simulink model "ScriptDemo"  (R2022b)
settings: configuration reference "TmVcThermal_Configuration_sub" (kept outside this file)
undefined symbols (not defined in the file or in its folder): aaaa, bbbb, cTmComprCtrl_D_u8HvacFlowTable_db, cTmComprCtrl_D_u8HvacFlowTable_sw, cTmComprCtrl_n_i16ChillCmpIMax, cTmComprCtrl_n_i16ChillCmpIMin, cTmComprCtrl_n_i16ChillCmpIMin666, cTmComprCtrl_n_i16ChillCmpPMax, cTmComprCtrl_n_i16ChillCmpPMin, cTmComprCtrl_n_i16CmpChillCoolRpmKiMax, cTmComprCtrl_n_i16CmpChillCoolRpmKiMin, cTmComprCtrl_n_i16CmpChillCoolRpmKpMax, cTmComprCtrl_n_i16CmpChillCoolRpmKpMin, cTmComprCtrl_n_i16CmpCoolRpmKiMax, cTmComprCtrl_n_i16CmpCoolRpmKiMin, cTmComprCtrl_n_i16CmpCoolRpmKpMax, cTmComprCtrl_n_i16CmpCoolRpmKpMin, cTmComprCtrl_n_i16SM4CmpHeatKiMax, cTmComprCtrl_n_i16SM4CmpHeatKiMin, cTmComprCtrl_n_i16SM4CmpHeatKpMax, cTmComprCtrl_n_i16SM4CmpHeatKpMin, cTmComprCtrl_n_i16SM5CmpHeatKiMax, cTmComprCtrl_n_i16SM5CmpHeatKiMin, cTmComprCtrl_n_i16SM5CmpHeatKpMax, cTmComprCtrl_n_i16SM5CmpHeatKpMin, cTmComprCtrl_n_i16SM6CmpHeatKiMax, cTmComprCtrl_n_i16SM6CmpHeatKiMin, cTmComprCtrl_n_i16SM6CmpHeatKpMax, cTmComprCtrl_n_i16SM6CmpHeatKpMin, cTmComprCtrl_n_u16CmpMaxSpdFanFltLimt, cTmComprCtrl_n_u16CmpMaxSpdLoSidePFltLimt, cTmComprCtrl_n_u16CmpMaxSpdSensorFltLimt, cTmComprCtrl_n_u16CompMinRpm, cTmComprCtrl_n_u16CompRpmIncThres, cTmComprCtrl_t_u16BattCooltFFPeriod, cTmComprCtrl_t_u16BattCooltPIPeriod, cTmComprCtrl_t_u16CmpCoolFFPeriod, cTmComprCtrl_t_u16CmpCoolPIPeriod, cTmComprCtrl_t_u16CoolCmpChillFFPeriod, cTmComprCtrl_t_u16CoolCmpChillPIPeriod, cTmComprCtrl_t_u16SM4CmpHeatFFPeriod, cTmComprCtrl_t_u16SM4CmpHeatPIPeriod, cTmComprCtrl_t_u16SM5CmpHeatFFPeriod, cTmComprCtrl_t_u16SM5CmpHeatPIPeriod, cTmComprCtrl_t_u16SM6CmpHeatFFPeriod, cTmComprCtrl_t_u16SM6CmpHeatPIPeriod, cTmComprCtrl_Te_EvapClearInteg, cTmComprCtrl_Te_i16HpReqTempSaturoffset, cTmComprCtrl_Te_i16SatLpReplaceDiff, cTmComprCtrl_Te_i16SM3BatDiffStartEvapDecOffset, cTmComprCtrl_Te_i16SM3EvapLo, cTmComprCtrl_Te_i16SM3TBatDiffEntEvapDecOffset, cTmComprCtrl_Te_i16SM3TBatDiffEntEvapDecOffsetQuit, cTmComprCtrl_Te_s32ErrCmpChillPIContinueCoolH, cTmComprCtrl_Te_s32ErrCmpChillPIContinueCoolL, cTmComprCtrl_Te_s32ErrCmpPIContinueChillH, cTmComprCtrl_Te_s32ErrCmpPIContinueChillL, cTmComprCtrl_Te_s32ErrCmpPIContinueCoolH, cTmComprCtrl_Te_s32ErrCmpPIContinueCoolL, cTmComprCtrl_Te_s32ErrCmpPIContinueHeatH ... (+398)
libraries: simulink x846, PCMULib x711, simulink_need_slupdate x4
(part 12 of 49)

== system ScriptDemo/Create/createSigOnLine/Before3 ==
  sTmRefriVlvCtrl_X_s32CEXVPosReqIn : Inport  OutDataTypeStr=single  OutputFunctionCall=on
  sTmRefriVlvCtrl_X_s32EEXVPosReqIn : Inport  Port=2  OutDataTypeStr=single
  sTmRefriVlvCtrl_X_s32BEXVPosReqIn : Inport  Port=3  OutDataTypeStr=single
  yTmRefriVlvCtrl_B_HpcCexvMovEnableIn : Inport  Port=4  OutDataTypeStr=boolean
  sTmRefriVlvCtrl_Z_u8CEXVInitStateIn : Inport  Port=5  OutDataTypeStr=uint8
  yTmRefriVlvCtrl_B_CexvCalibReqIn : Inport  Port=6  OutDataTypeStr=boolean
  yTmRefriVlvCtrl_B_HpcEexvMovEnableIn : Inport  Port=7  OutDataTypeStr=boolean
  sTmRefriVlvCtrl_Z_u8EEXVInitStateIn : Inport  Port=8  OutDataTypeStr=uint8
  yTmRefriVlvCtrl_B_EexvCalibReqIn : Inport  Port=9  OutDataTypeStr=boolean
  yTmRefriVlvCtrl_B_HpcBexvMovEnableIn : Inport  Port=10  OutDataTypeStr=boolean
  sTmRefriVlvCtrl_Z_u8BEXVInitStateIn : Inport  Port=11  OutDataTypeStr=uint8
  yTmRefriVlvCtrl_B_BexvCalibReqIn : Inport  Port=12  OutDataTypeStr=boolean
  sTmRefriVlvCtrl_X_s32SM3BexvMaxPosIn : Inport  Port=13  OutDataTypeStr=single
  yTmRefriVlvCtrl_B_EvapBattTLimBexvEnaIn : Inport  Port=14  OutDataTypeStr=boolean
  sTmRefriVlvCtrl_D_u8EexvRefriSwitchStIn : Inport  Port=15  OutDataTypeStr=uint8
  sTmRefriVlvCtrl_D_u8CexvRefriSwitchStIn : Inport  Port=16  OutDataTypeStr=uint8
  sTmRefriVlvCtrl_D_u8BexvRefriSwitchStIn : Inport  Port=17  OutDataTypeStr=uint8
  Before : Subsystem
  sTmRefriVlvCtrl_X_s32CEXVPosReq : Outport  OutDataTypeStr=single
  sTmRefriVlvCtrl_X_s32EEXVPosReq : Outport  Port=2  OutDataTypeStr=single
  sTmRefriVlvCtrl_X_s32BEXVPosReq : Outport  Port=3  OutDataTypeStr=single
  yTmRefriVlvCtrl_B_HpcCexvMovEnable : Outport  Port=4  OutDataTypeStr=boolean
  sTmRefriVlvCtrl_Z_u8CEXVInitState : Outport  Port=5  OutDataTypeStr=uint8
  yTmRefriVlvCtrl_B_CexvCalibReq : Outport  Port=6  OutDataTypeStr=boolean
  yTmRefriVlvCtrl_B_HpcEexvMovEnable : Outport  Port=7  OutDataTypeStr=boolean
  sTmRefriVlvCtrl_Z_u8EEXVInitState : Outport  Port=8  OutDataTypeStr=uint8
  yTmRefriVlvCtrl_B_EexvCalibReq : Outport  Port=9  OutDataTypeStr=boolean
  yTmRefriVlvCtrl_B_HpcBexvMovEnable : Outport  Port=10  OutDataTypeStr=boolean
  sTmRefriVlvCtrl_Z_u8BEXVInitState : Outport  Port=11  OutDataTypeStr=uint8
  yTmRefriVlvCtrl_B_BexvCalibReq : Outport  Port=12  OutDataTypeStr=boolean
  sTmRefriVlvCtrl_X_s32SM3BexvMaxPos : Outport  Port=13  OutDataTypeStr=single
  yTmRefriVlvCtrl_B_EvapBattTLimBexvEna : Outport  Port=14  OutDataTypeStr=boolean
  sTmRefriVlvCtrl_D_u8EexvRefriSwitchSt : Outport  Port=15  OutDataTypeStr=uint8
  sTmRefriVlvCtrl_D_u8CexvRefriSwitchSt : Outport  Port=16  OutDataTypeStr=uint8
  sTmRefriVlvCtrl_D_u8BexvRefriSwitchSt : Outport  Port=17  OutDataTypeStr=uint8
  wires:
  sTmRefriVlvCtrl_X_s32CEXVPosReqIn/1 -> Before/1(sTmRefriVlvCtrl_X_s32CEXVPosReqIn)
  sTmRefriVlvCtrl_X_s32EEXVPosReqIn/1 -> Before/2(sTmRefriVlvCtrl_X_s32EEXVPosReqIn)
  sTmRefriVlvCtrl_X_s32BEXVPosReqIn/1 -> Before/3(sTmRefriVlvCtrl_X_s32BEXVPosReqIn)
  yTmRefriVlvCtrl_B_HpcCexvMovEnableIn/1 -> Before/4(yTmRefriVlvCtrl_B_HpcCexvMovEnableIn)
  sTmRefriVlvCtrl_Z_u8CEXVInitStateIn/1 -> Before/5(sTmRefriVlvCtrl_Z_u8CEXVInitStateIn)
  yTmRefriVlvCtrl_B_CexvCalibReqIn/1 -> Before/6(yTmRefriVlvCtrl_B_CexvCalibReqIn)
  yTmRefriVlvCtrl_B_HpcEexvMovEnableIn/1 -> Before/7(yTmRefriVlvCtrl_B_HpcEexvMovEnableIn)
  sTmRefriVlvCtrl_Z_u8EEXVInitStateIn/1 -> Before/8(sTmRefriVlvCtrl_Z_u8EEXVInitStateIn)
  yTmRefriVlvCtrl_B_EexvCalibReqIn/1 -> Before/9(yTmRefriVlvCtrl_B_EexvCalibReqIn)
  yTmRefriVlvCtrl_B_HpcBexvMovEnableIn/1 -> Before/10(yTmRefriVlvCtrl_B_HpcBexvMovEnableIn)
  sTmRefriVlvCtrl_Z_u8BEXVInitStateIn/1 -> Before/11(sTmRefriVlvCtrl_Z_u8BEXVInitStateIn)
  yTmRefriVlvCtrl_B_BexvCalibReqIn/1 -> Before/12(yTmRefriVlvCtrl_B_BexvCalibReqIn)
  sTmRefriVlvCtrl_X_s32SM3BexvMaxPosIn/1 -> Before/13(sTmRefriVlvCtrl_X_s32SM3BexvMaxPosIn)
  yTmRefriVlvCtrl_B_EvapBattTLimBexvEnaIn/1 -> Before/14(yTmRefriVlvCtrl_B_EvapBattTLimBexvEnaIn)
  sTmRefriVlvCtrl_D_u8EexvRefriSwitchStIn/1 -> Before/15(sTmRefriVlvCtrl_D_u8EexvRefriSwitchStIn)
  sTmRefriVlvCtrl_D_u8CexvRefriSwitchStIn/1 -> Before/16(sTmRefriVlvCtrl_D_u8CexvRefriSwitchStIn)
  sTmRefriVlvCtrl_D_u8BexvRefriSwitchStIn/1 -> Before/17(sTmRefriVlvCtrl_D_u8BexvRefriSwitchStIn)
  Before/1(sTmRefriVlvCtrl_X_s32CEXVPosReq) -> sTmRefriVlvCtrl_X_s32CEXVPosReq/1
  Before/2(sTmRefriVlvCtrl_X_s32EEXVPosReq) -> sTmRefriVlvCtrl_X_s32EEXVPosReq/1
  Before/3(sTmRefriVlvCtrl_X_s32BEXVPosReq) -> sTmRefriVlvCtrl_X_s32BEXVPosReq/1
  Before/4(yTmRefriVlvCtrl_B_HpcCexvMovEnable) -> yTmRefriVlvCtrl_B_HpcCexvMovEnable/1
  Before/5(sTmRefriVlvCtrl_Z_u8CEXVInitState) -> sTmRefriVlvCtrl_Z_u8CEXVInitState/1
  Before/6(yTmRefriVlvCtrl_B_CexvCalibReq) -> yTmRefriVlvCtrl_B_CexvCalibReq/1
  Before/7(yTmRefriVlvCtrl_B_HpcEexvMovEnable) -> yTmRefriVlvCtrl_B_HpcEexvMovEnable/1
  Before/8(sTmRefriVlvCtrl_Z_u8EEXVInitState) -> sTmRefriVlvCtrl_Z_u8EEXVInitState/1
  Before/9(yTmRefriVlvCtrl_B_EexvCalibReq) -> yTmRefriVlvCtrl_B_EexvCalibReq/1
  Before/10(yTmRefriVlvCtrl_B_HpcBexvMovEnable) -> yTmRefriVlvCtrl_B_HpcBexvMovEnable/1
  Before/11(sTmRefriVlvCtrl_Z_u8BEXVInitState) -> sTmRefriVlvCtrl_Z_u8BEXVInitState/1
  Before/12(yTmRefriVlvCtrl_B_BexvCalibReq) -> yTmRefriVlvCtrl_B_BexvCalibReq/1
  Before/13(sTmRefriVlvCtrl_X_s32SM3BexvMaxPos) -> sTmRefriVlvCtrl_X_s32SM3BexvMaxPos/1
  Before/14(yTmRefriVlvCtrl_B_EvapBattTLimBexvEna) -> yTmRefriVlvCtrl_B_EvapBattTLimBexvEna/1
  Before/15(sTmRefriVlvCtrl_D_u8EexvRefriSwitchSt) -> sTmRefriVlvCtrl_D_u8EexvRefriSwitchSt/1
  Before/16(sTmRefriVlvCtrl_D_u8CexvRefriSwitchSt) -> sTmRefriVlvCtrl_D_u8CexvRefriSwitchSt/1
  Before/17(sTmRefriVlvCtrl_D_u8BexvRefriSwitchSt) -> sTmRefriVlvCtrl_D_u8BexvRefriSwitchSt/1

== system ScriptDemo/Create/createSigOnLine/Before4 ==
  sTmRefriVlvCtrl_X_s32CEXVPosReqIn : Inport  OutDataTypeStr=single  OutputFunctionCall=on
  sTmRefriVlvCtrl_X_s32EEXVPosReqIn : Inport  Port=2  OutDataTypeStr=single
  sTmRefriVlvCtrl_X_s32BEXVPosReqIn : Inport  Port=3  OutDataTypeStr=single
  yTmRefriVlvCtrl_B_HpcCexvMovEnableIn : Inport  Port=4  OutDataTypeStr=boolean
  sTmRefriVlvCtrl_Z_u8CEXVInitStateIn : Inport  Port=5  OutDataTypeStr=uint8
  yTmRefriVlvCtrl_B_CexvCalibReqIn : Inport  Port=6  OutDataTypeStr=boolean
  yTmRefriVlvCtrl_B_HpcEexvMovEnableIn : Inport  Port=7  OutDataTypeStr=boolean
  sTmRefriVlvCtrl_Z_u8EEXVInitStateIn : Inport  Port=8  OutDataTypeStr=uint8
  yTmRefriVlvCtrl_B_EexvCalibReqIn : Inport  Port=9  OutDataTypeStr=boolean
  yTmRefriVlvCtrl_B_HpcBexvMovEnableIn : Inport  Port=10  OutDataTypeStr=boolean
  sTmRefriVlvCtrl_Z_u8BEXVInitStateIn : Inport  Port=11  OutDataTypeStr=uint8
  yTmRefriVlvCtrl_B_BexvCalibReqIn : Inport  Port=12  OutDataTypeStr=boolean
  sTmRefriVlvCtrl_X_s32SM3BexvMaxPosIn : Inport  Port=13  OutDataTypeStr=single
  yTmRefriVlvCtrl_B_EvapBattTLimBexvEnaIn : Inport  Port=14  OutDataTypeStr=boolean
  sTmRefriVlvCtrl_D_u8EexvRefriSwitchStIn : Inport  Port=15  OutDataTypeStr=uint8
  sTmRefriVlvCtrl_D_u8CexvRefriSwitchStIn : Inport  Port=16  OutDataTypeStr=uint8
  sTmRefriVlvCtrl_D_u8BexvRefriSwitchStIn : Inport  Port=17  OutDataTypeStr=uint8
  Before : Subsystem
  sTmRefriVlvCtrl_X_s32CEXVPosReq : Outport  OutDataTypeStr=single
  sTmRefriVlvCtrl_X_s32EEXVPosReq : Outport  Port=2  OutDataTypeStr=single
  sTmRefriVlvCtrl_X_s32BEXVPosReq : Outport  Port=3  OutDataTypeStr=single
  yTmRefriVlvCtrl_B_HpcCexvMovEnable : Outport  Port=4  OutDataTypeStr=boolean
  sTmRefriVlvCtrl_Z_u8CEXVInitState : Outport  Port=5  OutDataTypeStr=uint8
  yTmRefriVlvCtrl_B_CexvCalibReq : Outport  Port=6  OutDataTypeStr=boolean
  yTmRefriVlvCtrl_B_HpcEexvMovEnable : Outport  Port=7  OutDataTypeStr=boolean
  sTmRefriVlvCtrl_Z_u8EEXVInitState : Outport  Port=8  OutDataTypeStr=uint8
  yTmRefriVlvCtrl_B_EexvCalibReq : Outport  Port=9  OutDataTypeStr=boolean
  yTmRefriVlvCtrl_B_HpcBexvMovEnable : Outport  Port=10  OutDataTypeStr=boolean
  sTmRefriVlvCtrl_Z_u8BEXVInitState : Outport  Port=11  OutDataTypeStr=uint8
  yTmRefriVlvCtrl_B_BexvCalibReq : Outport  Port=12  OutDataTypeStr=boolean
  sTmRefriVlvCtrl_X_s32SM3BexvMaxPos : Outport  Port=13  OutDataTypeStr=single
  yTmRefriVlvCtrl_B_EvapBattTLimBexvEna : Outport  Port=14  OutDataTypeStr=boolean
  sTmRefriVlvCtrl_D_u8EexvRefriSwitchSt : Outport  Port=15  OutDataTypeStr=uint8
  sTmRefriVlvCtrl_D_u8CexvRefriSwitchSt : Outport  Port=16  OutDataTypeStr=uint8
  sTmRefriVlvCtrl_D_u8BexvRefriSwitchSt : Outport  Port=17  OutDataTypeStr=uint8
  wires:
  sTmRefriVlvCtrl_X_s32CEXVPosReqIn/1 -> Before/1(sTmRefriVlvCtrl_X_s32CEXVPosReqIn)  "sTmRefriVlvCtrl_X_s32CEXVPosReqIn"
  sTmRefriVlvCtrl_X_s32EEXVPosReqIn/1 -> Before/2(sTmRefriVlvCtrl_X_s32EEXVPosReqIn)  "sTmRefriVlvCtrl_X_s32EEXVPosReqIn"
  sTmRefriVlvCtrl_X_s32BEXVPosReqIn/1 -> Before/3(sTmRefriVlvCtrl_X_s32BEXVPosReqIn)  "sTmRefriVlvCtrl_X_s32BEXVPosReqIn"
  yTmRefriVlvCtrl_B_HpcCexvMovEnableIn/1 -> Before/4(yTmRefriVlvCtrl_B_HpcCexvMovEnableIn)  "yTmRefriVlvCtrl_B_HpcCexvMovEnableIn"
  sTmRefriVlvCtrl_Z_u8CEXVInitStateIn/1 -> Before/5(sTmRefriVlvCtrl_Z_u8CEXVInitStateIn)  "sTmRefriVlvCtrl_Z_u8CEXVInitStateIn"
  yTmRefriVlvCtrl_B_CexvCalibReqIn/1 -> Before/6(yTmRefriVlvCtrl_B_CexvCalibReqIn)  "yTmRefriVlvCtrl_B_CexvCalibReqIn"
  yTmRefriVlvCtrl_B_HpcEexvMovEnableIn/1 -> Before/7(yTmRefriVlvCtrl_B_HpcEexvMovEnableIn)  "yTmRefriVlvCtrl_B_HpcEexvMovEnableIn"
  sTmRefriVlvCtrl_Z_u8EEXVInitStateIn/1 -> Before/8(sTmRefriVlvCtrl_Z_u8EEXVInitStateIn)  "sTmRefriVlvCtrl_Z_u8EEXVInitStateIn"
  yTmRefriVlvCtrl_B_EexvCalibReqIn/1 -> Before/9(yTmRefriVlvCtrl_B_EexvCalibReqIn)  "yTmRefriVlvCtrl_B_EexvCalibReqIn"
  yTmRefriVlvCtrl_B_HpcBexvMovEnableIn/1 -> Before/10(yTmRefriVlvCtrl_B_HpcBexvMovEnableIn)  "yTmRefriVlvCtrl_B_HpcBexvMovEnableIn"
  sTmRefriVlvCtrl_Z_u8BEXVInitStateIn/1 -> Before/11(sTmRefriVlvCtrl_Z_u8BEXVInitStateIn)  "sTmRefriVlvCtrl_Z_u8BEXVInitStateIn"
  yTmRefriVlvCtrl_B_BexvCalibReqIn/1 -> Before/12(yTmRefriVlvCtrl_B_BexvCalibReqIn)  "yTmRefriVlvCtrl_B_BexvCalibReqIn"
  sTmRefriVlvCtrl_X_s32SM3BexvMaxPosIn/1 -> Before/13(sTmRefriVlvCtrl_X_s32SM3BexvMaxPosIn)  "sTmRefriVlvCtrl_X_s32SM3BexvMaxPosIn"
  yTmRefriVlvCtrl_B_EvapBattTLimBexvEnaIn/1 -> Before/14(yTmRefriVlvCtrl_B_EvapBattTLimBexvEnaIn)  "yTmRefriVlvCtrl_B_EvapBattTLimBexvEnaIn"
  sTmRefriVlvCtrl_D_u8EexvRefriSwitchStIn/1 -> Before/15(sTmRefriVlvCtrl_D_u8EexvRefriSwitchStIn)  "sTmRefriVlvCtrl_D_u8EexvRefriSwitchStIn"
  sTmRefriVlvCtrl_D_u8CexvRefriSwitchStIn/1 -> Before/16(sTmRefriVlvCtrl_D_u8CexvRefriSwitchStIn)  "sTmRefriVlvCtrl_D_u8CexvRefriSwitchStIn"
  sTmRefriVlvCtrl_D_u8BexvRefriSwitchStIn/1 -> Before/17(sTmRefriVlvCtrl_D_u8BexvRefriSwitchStIn)  "sTmRefriVlvCtrl_D_u8BexvRefriSwitchStIn"
  Before/1(sTmRefriVlvCtrl_X_s32CEXVPosReq) -> sTmRefriVlvCtrl_X_s32CEXVPosReq/1
  Before/2(sTmRefriVlvCtrl_X_s32EEXVPosReq) -> sTmRefriVlvCtrl_X_s32EEXVPosReq/1
  Before/3(sTmRefriVlvCtrl_X_s32BEXVPosReq) -> sTmRefriVlvCtrl_X_s32BEXVPosReq/1
  Before/4(yTmRefriVlvCtrl_B_HpcCexvMovEnable) -> yTmRefriVlvCtrl_B_HpcCexvMovEnable/1
  Before/5(sTmRefriVlvCtrl_Z_u8CEXVInitState) -> sTmRefriVlvCtrl_Z_u8CEXVInitState/1
  Before/6(yTmRefriVlvCtrl_B_CexvCalibReq) -> yTmRefriVlvCtrl_B_CexvCalibReq/1
  Before/7(yTmRefriVlvCtrl_B_HpcEexvMovEnable) -> yTmRefriVlvCtrl_B_HpcEexvMovEnable/1
  Before/8(sTmRefriVlvCtrl_Z_u8EEXVInitState) -> sTmRefriVlvCtrl_Z_u8EEXVInitState/1
  Before/9(yTmRefriVlvCtrl_B_EexvCalibReq) -> yTmRefriVlvCtrl_B_EexvCalibReq/1
  Before/10(yTmRefriVlvCtrl_B_HpcBexvMovEnable) -> yTmRefriVlvCtrl_B_HpcBexvMovEnable/1
  Before/11(sTmRefriVlvCtrl_Z_u8BEXVInitState) -> sTmRefriVlvCtrl_Z_u8BEXVInitState/1
  Before/12(yTmRefriVlvCtrl_B_BexvCalibReq) -> yTmRefriVlvCtrl_B_BexvCalibReq/1
  Before/13(sTmRefriVlvCtrl_X_s32SM3BexvMaxPos) -> sTmRefriVlvCtrl_X_s32SM3BexvMaxPos/1
  Before/14(yTmRefriVlvCtrl_B_EvapBattTLimBexvEna) -> yTmRefriVlvCtrl_B_EvapBattTLimBexvEna/1
  Before/15(sTmRefriVlvCtrl_D_u8EexvRefriSwitchSt) -> sTmRefriVlvCtrl_D_u8EexvRefriSwitchSt/1
  Before/16(sTmRefriVlvCtrl_D_u8CexvRefriSwitchSt) -> sTmRefriVlvCtrl_D_u8CexvRefriSwitchSt/1
  Before/17(sTmRefriVlvCtrl_D_u8BexvRefriSwitchSt) -> sTmRefriVlvCtrl_D_u8BexvRefriSwitchSt/1

== system ScriptDemo/Create/createStoreMem/After ==
  DataStoreMemory : DataStoreMemory  DataStoreName=cTmRefriVlvCtrl_n_u16BexvLmtCompSpdOffset  InitialValue=100  ShowAdditionalParam=off  OutDataTypeStr=uint16
  DataStoreMemory1 : DataStoreMemory  DataStoreName=cTmRefriVlvCtrl_p_u16BexvKeepHPres  InitialValue=2800  ShowAdditionalParam=off  OutDataTypeStr=uint16
  DataStoreMemory10 : DataStoreMemory  DataStoreName=cTmRefriVlvCtrl_Te_s16SCCurDiffSM4CEXVPI  ShowAdditionalParam=off  OutDataTypeStr=int16
  DataStoreMemory11 : DataStoreMemory  DataStoreName=cTmRefriVlvCtrl_Te_s32BexvKeepTDischarge  InitialValue=120  ShowAdditionalParam=off  OutDataTypeStr=single
  DataStoreMemory12 : DataStoreMemory  DataStoreName=cTmRefriVlvCtrl_Te_s32EvapProtect  InitialValue=1.5  ShowAdditionalParam=off  OutDataTypeStr=single
  DataStoreMemory13 : DataStoreMemory  DataStoreName=cTmRefriVlvCtrl_Te_s32EvapProtectRecover  InitialValue=3  ShowAdditionalParam=off  OutDataTypeStr=single
  DataStoreMemory14 : DataStoreMemory  DataStoreName=cTmRefriVlvCtrl_Te_s32SM1SHHigh  InitialValue=20  ShowAdditionalParam=off  OutDataTypeStr=single
  DataStoreMemory2 : DataStoreMemory  DataStoreName=cTmRefriVlvCtrl_p_u16SM4CexvHiDischarge  InitialValue=115  ShowAdditionalParam=off  OutDataTypeStr=uint16
  DataStoreMemory3 : DataStoreMemory  DataStoreName=cTmRefriVlvCtrl_p_u16SM4CexvHiPres  InitialValue=2800  ShowAdditionalParam=off  OutDataTypeStr=uint16
  DataStoreMemory4 : DataStoreMemory  DataStoreName=cTmRefriVlvCtrl_p_u16SM6CexvHiDischarge  InitialValue=115  ShowAdditionalParam=off  OutDataTypeStr=uint16
  DataStoreMemory5 : DataStoreMemory  DataStoreName=cTmRefriVlvCtrl_p_u16SM6CexvHiPres  InitialValue=2800  ShowAdditionalParam=off  OutDataTypeStr=uint16
  DataStoreMemory6 : DataStoreMemory  DataStoreName=cTmRefriVlvCtrl_t_s32BexvPosnCalibReqTime  InitialValue=2  ShowAdditionalParam=off  OutDataTypeStr=single
  DataStoreMemory7 : DataStoreMemory  DataStoreName=cTmRefriVlvCtrl_t_s32CexvPosnCalibReqTime  InitialValue=2  ShowAdditionalParam=off  OutDataTypeStr=single
  DataStoreMemory8 : DataStoreMemory  DataStoreName=cTmRefriVlvCtrl_t_s32EexvPosnCalibReqTime  InitialValue=2  ShowAdditionalParam=off  OutDataTypeStr=single
  DataStoreMemory9 : DataStoreMemory  DataStoreName=cTmRefriVlvCtrl_t_s32SM0DecPreTime  InitialValue=1  ShowAdditionalParam=off  OutDataTypeStr=single
  DataStoreWrite : DataStoreWrite  DataStoreName=cTmRefriVlvCtrl_n_u16BexvLmtCompSpdOffset  IndexOptions=Index vector (dialog)  Indices=1  OutputSizes=1
  DataStoreWrite1 : DataStoreWrite  DataStoreName=cTmRefriVlvCtrl_p_u16BexvKeepHPres  IndexOptions=Index vector (dialog)  Indices=1  OutputSizes=1
  DataStoreWrite10 : DataStoreWrite  DataStoreName=cTmRefriVlvCtrl_Te_s16SCCurDiffSM4CEXVPI  IndexOptions=Index vector (dialog)  Indices=1  OutputSizes=1
  DataStoreWrite11 : DataStoreWrite  DataStoreName=cTmRefriVlvCtrl_Te_s32BexvKeepTDischarge  IndexOptions=Index vector (dialog)  Indices=1  OutputSizes=1
  DataStoreWrite12 : DataStoreWrite  DataStoreName=cTmRefriVlvCtrl_Te_s32EvapProtect  IndexOptions=Index vector (dialog)  Indices=1  OutputSizes=1
  DataStoreWrite13 : DataStoreWrite  DataStoreName=cTmRefriVlvCtrl_Te_s32EvapProtectRecover  IndexOptions=Index vector (dialog)  Indices=1  OutputSizes=1
  DataStoreWrite14 : DataStoreWrite  DataStoreName=cTmRefriVlvCtrl_Te_s32SM1SHHigh  IndexOptions=Index vector (dialog)  Indices=1  OutputSizes=1
  DataStoreWrite2 : DataStoreWrite  DataStoreName=cTmRefriVlvCtrl_p_u16SM4CexvHiDischarge  IndexOptions=Index vector (dialog)  Indices=1  OutputSizes=1
  DataStoreWrite3 : DataStoreWrite  DataStoreName=cTmRefriVlvCtrl_p_u16SM4CexvHiPres  IndexOptions=Index vector (dialog)  Indices=1  OutputSizes=1
  DataStoreWrite4 : DataStoreWrite  DataStoreName=cTmRefriVlvCtrl_p_u16SM6CexvHiDischarge  IndexOptions=Index vector (dialog)  Indices=1  OutputSizes=1
  DataStoreWrite5 : DataStoreWrite  DataStoreName=cTmRefriVlvCtrl_p_u16SM6CexvHiPres  IndexOptions=Index vector (dialog)  Indices=1  OutputSizes=1
  DataStoreWrite6 : DataStoreWrite  DataStoreName=cTmRefriVlvCtrl_t_s32BexvPosnCalibReqTime  IndexOptions=Index vector (dialog)  Indices=1  OutputSizes=1
  DataStoreWrite7 : DataStoreWrite  DataStoreName=cTmRefriVlvCtrl_t_s32CexvPosnCalibReqTime  IndexOptions=Index vector (dialog)  Indices=1  OutputSizes=1
  DataStoreWrite8 : DataStoreWrite  DataStoreName=cTmRefriVlvCtrl_t_s32EexvPosnCalibReqTime  IndexOptions=Index vector (dialog)  Indices=1  OutputSizes=1
  DataStoreWrite9 : DataStoreWrite  DataStoreName=cTmRefriVlvCtrl_t_s32SM0DecPreTime  IndexOptions=Index vector (dialog)  Indices=1  OutputSizes=1
  MultiPortSwitch : MultiPortSwitch  Inputs=15
  ReadcTmRefriVlvCtrl_Te_s16SCCurDiffSM4CEXVPI : DataStoreRead  DataStoreName=cTmRefriVlvCtrl_Te_s16SCCurDiffSM4CEXVPI  IndexOptions=Index vector (dialog)  Indices=1  OutputSizes=1
  ReadcTmRefriVlvCtrl_Te_s32BexvKeepTDischarge : DataStoreRead  DataStoreName=cTmRefriVlvCtrl_Te_s32BexvKeepTDischarge  IndexOptions=Index vector (dialog)  Indices=1  OutputSizes=1
  ReadcTmRefriVlvCtrl_Te_s32EvapProtect : DataStoreRead  DataStoreName=cTmRefriVlvCtrl_Te_s32EvapProtect  IndexOptions=Index vector (dialog)  Indices=1  OutputSizes=1
  ReadcTmRefriVlvCtrl_Te_s32EvapProtectRecover : DataStoreRead  DataStoreName=cTmRefriVlvCtrl_Te_s32EvapProtectRecover  IndexOptions=Index vector (dialog)  Indices=1  OutputSizes=1
  ReadcTmRefriVlvCtrl_Te_s32SM1SHHigh : DataStoreRead  DataStoreName=cTmRefriVlvCtrl_Te_s32SM1SHHigh  IndexOptions=Index vector (dialog)  Indices=1  OutputSizes=1
  ReadcTmRefriVlvCtrl_n_u16BexvLmtCompSpdOffset : DataStoreRead  DataStoreName=cTmRefriVlvCtrl_n_u16BexvLmtCompSpdOffset  IndexOptions=Index vector (dialog)  Indices=1  OutputSizes=1
  ReadcTmRefriVlvCtrl_p_u16BexvKeepHPres : DataStoreRead  DataStoreName=cTmRefriVlvCtrl_p_u16BexvKeepHPres  IndexOptions=Index vector (dialog)  Indices=1  OutputSizes=1
  ReadcTmRefriVlvCtrl_p_u16SM4CexvHiDischarge : DataStoreRead  DataStoreName=cTmRefriVlvCtrl_p_u16SM4CexvHiDischarge  IndexOptions=Index vector (dialog)  Indices=1  OutputSizes=1
  ReadcTmRefriVlvCtrl_p_u16SM4CexvHiPres : DataStoreRead  DataStoreName=cTmRefriVlvCtrl_p_u16SM4CexvHiPres  IndexOptions=Index vector (dialog)  Indices=1  OutputSizes=1
  ReadcTmRefriVlvCtrl_p_u16SM6CexvHiDischarge : DataStoreRead  DataStoreName=cTmRefriVlvCtrl_p_u16SM6CexvHiDischarge  IndexOptions=Index vector (dialog)  Indices=1  OutputSizes=1
  ReadcTmRefriVlvCtrl_p_u16SM6CexvHiPres : DataStoreRead  DataStoreName=cTmRefriVlvCtrl_p_u16SM6CexvHiPres  IndexOptions=Index vector (dialog)  Indices=1  OutputSizes=1
  ReadcTmRefriVlvCtrl_t_s32BexvPosnCalibReqTime : DataStoreRead  DataStoreName=cTmRefriVlvCtrl_t_s32BexvPosnCalibReqTime  IndexOptions=Index vector (dialog)  Indices=1  OutputSizes=1
  ReadcTmRefriVlvCtrl_t_s32CexvPosnCalibReqTime : DataStoreRead  DataStoreName=cTmRefriVlvCtrl_t_s32CexvPosnCalibReqTime  IndexOptions=Index vector (dialog)  Indices=1  OutputSizes=1
  ReadcTmRefriVlvCtrl_t_s32EexvPosnCalibReqTime : DataStoreRead  DataStoreName=cTmRefriVlvCtrl_t_s32EexvPosnCalibReqTime  IndexOptions=Index vector (dialog)  Indices=1  OutputSizes=1
  ReadcTmRefriVlvCtrl_t_s32SM0DecPreTime : DataStoreRead  DataStoreName=cTmRefriVlvCtrl_t_s32SM0DecPreTime  IndexOptions=Index vector (dialog)  Indices=1  OutputSizes=1
  cTmRefriVlvCtrl_Te_s16SCCurDiffSM4CEXVPI : DisplayBlock  LabelPosition=Hide
  cTmRefriVlvCtrl_Te_s32BexvKeepTDischarge : DisplayBlock  LabelPosition=Hide
  cTmRefriVlvCtrl_Te_s32EvapProtect : DisplayBlock  LabelPosition=Hide
  cTmRefriVlvCtrl_Te_s32EvapProtectRecover : DisplayBlock  LabelPosition=Hide
  cTmRefriVlvCtrl_Te_s32SM1SHHigh : DisplayBlock  LabelPosition=Hide
  cTmRefriVlvCtrl_n_u16BexvLmtCompSpdOffset : DisplayBlock  LabelPosition=Hide
  cTmRefriVlvCtrl_p_u16BexvKeepHPres : DisplayBlock  LabelPosition=Hide
  cTmRefriVlvCtrl_p_u16SM4CexvHiDischarge : DisplayBlock  LabelPosition=Hide
  cTmRefriVlvCtrl_p_u16SM4CexvHiPres : DisplayBlock  LabelPosition=Hide
  cTmRefriVlvCtrl_p_u16SM6CexvHiDischarge : DisplayBlock  LabelPosition=Hide
  cTmRefriVlvCtrl_p_u16SM6CexvHiPres : DisplayBlock  LabelPosition=Hide
  cTmRefriVlvCtrl_t_s32BexvPosnCalibReqTime : DisplayBlock  LabelPosition=Hide
  cTmRefriVlvCtrl_t_s32CexvPosnCalibReqTime : DisplayBlock  LabelPosition=Hide
  cTmRefriVlvCtrl_t_s32EexvPosnCalibReqTime : DisplayBlock  LabelPosition=Hide
  cTmRefriVlvCtrl_t_s32SM0DecPreTime : DisplayBlock  LabelPosition=Hide
  wires:
  ReadcTmRefriVlvCtrl_n_u16BexvLmtCompSpdOffset/1 -> MultiPortSwitch/2
  ReadcTmRefriVlvCtrl_p_u16BexvKeepHPres/1 -> MultiPortSwitch/3
  ReadcTmRefriVlvCtrl_p_u16SM4CexvHiDischarge/1 -> MultiPortSwitch/4
  ReadcTmRefriVlvCtrl_p_u16SM4CexvHiPres/1 -> MultiPortSwitch/5
  ReadcTmRefriVlvCtrl_p_u16SM6CexvHiDischarge/1 -> MultiPortSwitch/6
  ReadcTmRefriVlvCtrl_p_u16SM6CexvHiPres/1 -> MultiPortSwitch/7
  ReadcTmRefriVlvCtrl_t_s32BexvPosnCalibReqTime/1 -> MultiPortSwitch/8
  ReadcTmRefriVlvCtrl_t_s32CexvPosnCalibReqTime/1 -> MultiPortSwitch/9
  ReadcTmRefriVlvCtrl_t_s32EexvPosnCalibReqTime/1 -> MultiPortSwitch/10
  ReadcTmRefriVlvCtrl_t_s32SM0DecPreTime/1 -> MultiPortSwitch/11
  ReadcTmRefriVlvCtrl_Te_s16SCCurDiffSM4CEXVPI/1 -> MultiPortSwitch/12
  ReadcTmRefriVlvCtrl_Te_s32BexvKeepTDischarge/1 -> MultiPortSwitch/13
  ReadcTmRefriVlvCtrl_Te_s32EvapProtect/1 -> MultiPortSwitch/14
  ReadcTmRefriVlvCtrl_Te_s32EvapProtectRecover/1 -> MultiPortSwitch/15
  ReadcTmRefriVlvCtrl_Te_s32SM1SHHigh/1 -> MultiPortSwitch/16

== system ScriptDemo/Create/createSubMod/After ==
  Fun666666_Req26245_DemoSub1 : Subsystem
  Fun666666_Req26246_DemoSub2 : Subsystem
  Fun666666_Req26247_DemoSub3 : Subsystem
  Fun666666_Req26248_DemoSub4 : Subsystem
  Fun666666_Req26249_DemoSub5 : Subsystem
  Fun888888_Req26250_DemoSub6 : Subsystem
  Fun888888_Req26251_DemoSub7 : Subsystem
  Fun888888_Req26252_DemoSub8 : Subsystem
  Fun888888_Req26253_DemoSub9 : Subsystem
  Fun888888_Req26254_DemoSub10 : Subsystem

== system ScriptDemo/Create/createSubmodInfo/After ==
  note: <模型信息: After>
      |
      |
      | 【输入端口】
      | 1. sTmSigProces_D_u8BattThermReq
      | 2. sTmIn_D_u8DCChrgSt
      | 3. sTmSigProces_D_u8HvBattCoolgReq
      | 4. rTmComprCtrl_Te_s32TempError
      |
      | 【输出端口】
      | 1. SM1Kp
      |
      | 【标定量】
      | 1. cTmComprCtrl_n_u16CompRpmIncThres=3000
      | 2. mTmComprCtrl_n_u16KpBattCooltRpmCharging
      | 3. mTmComprCtrl_n_u16KpBattCooltRpmCharging_X
      | 4. mTmComprCtrl_n_u16KpBattCooltRpmCharging_Y
      | 5. mTmComprCtrl_n_u16KpBattCooltRpmNorm
      | 6. mTmComprCtrl_n_u16KpBattCooltRpmNorm_X
      | 7. mTmComprCtrl_n_u16KpBattCooltRpmNorm_Y
      | 8. mTmComprCtrl_n_u16KpBattCooltRpmSuperCharging
      | 9. mTmComprCtrl_n_u16KpBattCooltRpmSuperCharging_X
      | 10. mTmComprCtrl_n_u16KpBattCooltRpmSuperCharging_Y
      |
      | 创建时间: 2025-04-15 14:34:45
  sTmSigProces_D_u8BattThermReq : Inport
  sTmIn_D_u8DCChrgSt : Inport  Port=2
  sTmSigProces_D_u8HvBattCoolgReq : Inport  Port=3
  rTmComprCtrl_Te_s32TempError : Inport  Port=4
  2-D Lookup Table5 : Lookup_n-D  LookupTableObject=mTmComprCtrl_n_u16FFBattCooltRpmCharging  BreakpointsForDimension1=mTmComprCtrl_n_u16KpBattCooltRpmNorm_Y  BreakpointsForDimension2=mTmComprCtrl_n_u16KpBattCooltRpmNorm_X  BreakpointsForDimension1DataTypeStr=Inherit: Inherit from 'Breakpoint data'  BreakpointsForDimension2DataTypeStr=Inherit: Inherit from 'Breakpoint data'  Table=mTmComprCtrl_n_u16KpBattCooltRpmNorm  TableDataTypeStr=Inherit: Inherit from 'Table data'  ExtrapMethod=Clip  InternalRulePriority=Speed  OutDataTypeStr=Inherit: Inherit via back propagation  RndMeth=Simplest  InputSameDT=off
      settings: InputPortMap=u0,u1
  2-D Lookup Table6 : Lookup_n-D  LookupTableObject=mTmComprCtrl_n_u16FFBattCooltRpmCharging  BreakpointsForDimension1=mTmComprCtrl_n_u16KpBattCooltRpmCharging_Y  BreakpointsForDimension2=mTmComprCtrl_n_u16KpBattCooltRpmCharging_X  BreakpointsForDimension1DataTypeStr=Inherit: Inherit from 'Breakpoint data'  BreakpointsForDimension2DataTypeStr=Inherit: Inherit from 'Breakpoint data'  Table=mTmComprCtrl_n_u16KpBattCooltRpmCharging  TableDataTypeStr=Inherit: Inherit from 'Table data'  ExtrapMethod=Clip  InternalRulePriority=Speed  OutDataTypeStr=Inherit: Inherit via back propagation  RndMeth=Simplest  InputSameDT=off
      settings: InputPortMap=u0,u1
  2-D Lookup Table7 : Lookup_n-D  LookupTableObject=mTmComprCtrl_n_u16FFBattCooltRpmCharging  BreakpointsForDimension1=mTmComprCtrl_n_u16KpBattCooltRpmSuperCharging_Y  BreakpointsForDimension2=mTmComprCtrl_n_u16KpBattCooltRpmSuperCharging_X  BreakpointsForDimension1DataTypeStr=Inherit: Inherit from 'Breakpoint data'  BreakpointsForDimension2DataTypeStr=Inherit: Inherit from 'Breakpoint data'  Table=mTmComprCtrl_n_u16KpBattCooltRpmSuperCharging  TableDataTypeStr=Inherit: Inherit from 'Table data'  ExtrapMethod=Clip  InternalRulePriority=Speed  OutDataTypeStr=Inherit: Inherit via back propagation  RndMeth=Simplest  InputSameDT=off
      settings: InputPortMap=u0,u1
  Constant : Constant  Value=cTmComprCtrl_n_u16CompRpmIncThres
  Terminator : Terminator
  tableChoose : Subsystem
  SM1Kp : Outport
  wires:
  sTmIn_D_u8DCChrgSt/1 -> tableChoose/2(sTmIn_D_u8DCChrgSt)
  sTmSigProces_D_u8BattThermReq/1 -> tableChoose/1(sTmSigProces_D_u8BattThermReq)
  2-D Lookup Table7/1 -> tableChoose/5(tab3)
  2-D Lookup Table5/1 -> tableChoose/3(tab1)
  2-D Lookup Table6/1 -> tableChoose/4(tab2)
  sTmSigProces_D_u8HvBattCoolgReq/1 -> 2-D Lookup Table7/1, 2-D Lookup Table6/1, 2-D Lookup Table5/1
  rTmComprCtrl_Te_s32TempError/1 -> 2-D Lookup Table7/2, 2-D Lookup Table6/2, 2-D Lookup Table5/2
  tableChoose/1(out) -> SM1Kp/1
  Constant/1 -> Terminator/1

== system ScriptDemo/Create/createSubmodInfo/Before ==
  sTmSigProces_D_u8BattThermReq : Inport
  sTmIn_D_u8DCChrgSt : Inport  Port=2
  sTmSigProces_D_u8HvBattCoolgReq : Inport  Port=3
  rTmComprCtrl_Te_s32TempError : Inport  Port=4
  2-D Lookup Table5 : Lookup_n-D  LookupTableObject=mTmComprCtrl_n_u16FFBattCooltRpmCharging  BreakpointsForDimension1=mTmComprCtrl_n_u16KpBattCooltRpmNorm_Y  BreakpointsForDimension2=mTmComprCtrl_n_u16KpBattCooltRpmNorm_X  BreakpointsForDimension1DataTypeStr=Inherit: Inherit from 'Breakpoint data'  BreakpointsForDimension2DataTypeStr=Inherit: Inherit from 'Breakpoint data'  Table=mTmComprCtrl_n_u16KpBattCooltRpmNorm  TableDataTypeStr=Inherit: Inherit from 'Table data'  ExtrapMethod=Clip  InternalRulePriority=Speed  OutDataTypeStr=Inherit: Inherit via back propagation  RndMeth=Simplest  InputSameDT=off
      settings: InputPortMap=u0,u1
  2-D Lookup Table6 : Lookup_n-D  LookupTableObject=mTmComprCtrl_n_u16FFBattCooltRpmCharging  BreakpointsForDimension1=mTmComprCtrl_n_u16KpBattCooltRpmCharging_Y  BreakpointsForDimension2=mTmComprCtrl_n_u16KpBattCooltRpmCharging_X  BreakpointsForDimension1DataTypeStr=Inherit: Inherit from 'Breakpoint data'  BreakpointsForDimension2DataTypeStr=Inherit: Inherit from 'Breakpoint data'  Table=mTmComprCtrl_n_u16KpBattCooltRpmCharging  TableDataTypeStr=Inherit: Inherit from 'Table data'  ExtrapMethod=Clip  InternalRulePriority=Speed  OutDataTypeStr=Inherit: Inherit via back propagation  RndMeth=Simplest  InputSameDT=off
      settings: InputPortMap=u0,u1
  2-D Lookup Table7 : Lookup_n-D  LookupTableObject=mTmComprCtrl_n_u16FFBattCooltRpmCharging  BreakpointsForDimension1=mTmComprCtrl_n_u16KpBattCooltRpmSuperCharging_Y  BreakpointsForDimension2=mTmComprCtrl_n_u16KpBattCooltRpmSuperCharging_X  BreakpointsForDimension1DataTypeStr=Inherit: Inherit from 'Breakpoint data'  BreakpointsForDimension2DataTypeStr=Inherit: Inherit from 'Breakpoint data'  Table=mTmComprCtrl_n_u16KpBattCooltRpmSuperCharging  TableDataTypeStr=Inherit: Inherit from 'Table data'  ExtrapMethod=Clip  InternalRulePriority=Speed  OutDataTypeStr=Inherit: Inherit via back propagation  RndMeth=Simplest  InputSameDT=off
      settings: InputPortMap=u0,u1
  tableChoose : Subsystem
  SM1Kp : Outport
  wires:
  sTmIn_D_u8DCChrgSt/1 -> tableChoose/2(sTmIn_D_u8DCChrgSt)
  sTmSigProces_D_u8BattThermReq/1 -> tableChoose/1(sTmSigProces_D_u8BattThermReq)
  2-D Lookup Table7/1 -> tableChoose/5(tab3)
  2-D Lookup Table5/1 -> tableChoose/3(tab1)
  2-D Lookup Table6/1 -> tableChoose/4(tab2)
  sTmSigProces_D_u8HvBattCoolgReq/1 -> 2-D Lookup Table7/1, 2-D Lookup Table6/1, 2-D Lookup Table5/1
  rTmComprCtrl_Te_s32TempError/1 -> 2-D Lookup Table7/2, 2-D Lookup Table6/2, 2-D Lookup Table5/2
  tableChoose/1(out) -> SM1Kp/1

== system ScriptDemo/Create/createSwitchCase/After ==
  note: %% 输入参数处理
      | p = inputParser; % 函数的输入解析器
      | addParameter(p, 'caseList' , '{1,2,3,[4 5 6]}' ); % case 的输入值
      | addParameter(p, 'caseIn' , 'Demo' ); % case 输入信号
      | addParameter(p, 'caseNames' , ...
      | { 'rTmComprCtrl_Te_s32TempError' , 'rTmComprCtrl_n_u16ComprRpmFF' , ...
      | 'rTmComprCtrl_n_u16ComprRpmKp' , 'rTmComprCtrl_n_u16ComprRpmKi' , ...
      | }); % case 具体名称列表
      | addParameter(p, 'sigNames' , ...
      | { 'demo1' , 'demo2' }); % switch 的输出信号
      | addParameter(p, 'actionPosYShift' ,50); % 每个case 的偏移值
      | addParameter(p, 'caseGap' ,30); % switch case 的间距
      | addParameter(p, 'caseStp' ,1); % switch case 间距放大系数
      | addParameter(p, 'resovleSig' ,true); % 经过merge后，是否需要解析信号
      |
      | createSwitchCase( ...
      | 'caseIn' , 'sTmRefriModeMgr_D_u8ModeSwitchType' , ...
      | 'caseList' , '{1,17,[8 9 10 11 12 13 18 19],20,21,22,23}' , ...
      | 'caseNames' ,{ 'Stop' , 'HoldSwitch' , 'ReduceRpm' , 'Test' , 'Test2' , 'Test3' , 'Test4' }, ...
      | 'sigNames' ,{ 'xTmComprCtrl_B_ChangeFinished' , 'rTmComprCtrl_n_u16CompRpmReq' })
  Default : Subsystem  TreatAsAtomicUnit=on
  HoldSwitch : Subsystem  TreatAsAtomicUnit=on
  Merge : Merge  Inputs=8
  Merge1 : Merge  Inputs=8
  ReduceRpm : Subsystem  TreatAsAtomicUnit=on
  Stop : Subsystem  TreatAsAtomicUnit=on
  Switch Case : SwitchCase  CaseConditions={1,17,[8 9 10 11 12 13 18 19],20,21,22,23}
  Test : Subsystem  TreatAsAtomicUnit=on
  Test2 : Subsystem  TreatAsAtomicUnit=on
  Test3 : Subsystem  TreatAsAtomicUnit=on
  Test4 : Subsystem  TreatAsAtomicUnit=on
  wires:
  [sTmRefriModeMgr_D_u8ModeSwitchType] -> Switch Case/1
  [Stop] -> Stop/Action
  [HoldSwitch] -> HoldSwitch/Action
  [ReduceRpm] -> ReduceRpm/Action
  [Test] -> Test/Action
  [Test2] -> Test2/Action
  [Test3] -> Test3/Action
  [Test4] -> Test4/Action
  [Default] -> Default/Action
  [xDefault_B_ChangeFinished] -> Merge/1
  [xHoldSwitch_B_ChangeFinished] -> Merge/2
  [xReduceRpm_B_ChangeFinished] -> Merge/3
  [xStop_B_ChangeFinished] -> Merge/4
  [xTest_B_ChangeFinished] -> Merge/5
  [xTest2_B_ChangeFinished] -> Merge/6
  [xTest3_B_ChangeFinished] -> Merge/7
  [xTest4_B_ChangeFinished] -> Merge/8
  Merge/1 -> [xTmComprCtrl_B_ChangeFinished]  "xTmComprCtrl_B_ChangeFinished"
  [rDefault_n_u16CompRpmReq] -> Merge1/1
  [rHoldSwitch_n_u16CompRpmReq] -> Merge1/2
  [rReduceRpm_n_u16CompRpmReq] -> Merge1/3
  [rStop_n_u16CompRpmReq] -> Merge1/4
  [rTest_n_u16CompRpmReq] -> Merge1/5
  [rTest2_n_u16CompRpmReq] -> Merge1/6
  [rTest3_n_u16CompRpmReq] -> Merge1/7
  [rTest4_n_u16CompRpmReq] -> Merge1/8
  Merge1/1 -> [rTmComprCtrl_n_u16CompRpmReq]  "rTmComprCtrl_n_u16CompRpmReq"
  Default/1(xDefault_B_ChangeFinished) -> [xDefault_B_ChangeFinished]
  Default/2(rDefault_n_u16CompRpmReq) -> [rDefault_n_u16CompRpmReq]
  HoldSwitch/1(xHoldSwitch_B_ChangeFinished) -> [xHoldSwitch_B_ChangeFinished]
  HoldSwitch/2(rHoldSwitch_n_u16CompRpmReq) -> [rHoldSwitch_n_u16CompRpmReq]
  ReduceRpm/1(xReduceRpm_B_ChangeFinished) -> [xReduceRpm_B_ChangeFinished]
  ReduceRpm/2(rReduceRpm_n_u16CompRpmReq) -> [rReduceRpm_n_u16CompRpmReq]
  Stop/1(xStop_B_ChangeFinished) -> [xStop_B_ChangeFinished]
  Stop/2(rStop_n_u16CompRpmReq) -> [rStop_n_u16CompRpmReq]
  Test/1(xTest_B_ChangeFinished) -> [xTest_B_ChangeFinished]
  Test/2(rTest_n_u16CompRpmReq) -> [rTest_n_u16CompRpmReq]
  Test2/1(xTest2_B_ChangeFinished) -> [xTest2_B_ChangeFinished]
  Test2/2(rTest2_n_u16CompRpmReq) -> [rTest2_n_u16CompRpmReq]
  Test3/1(xTest3_B_ChangeFinished) -> [xTest3_B_ChangeFinished]
  Test3/2(rTest3_n_u16CompRpmReq) -> [rTest3_n_u16CompRpmReq]
  Test4/1(xTest4_B_ChangeFinished) -> [xTest4_B_ChangeFinished]
  Test4/2(rTest4_n_u16CompRpmReq) -> [rTest4_n_u16CompRpmReq]

== system ScriptDemo/Delete/delUselessLine/After ==
  In1 : Inport
  In2 : Inport  Port=2
  In3 : Inport  Port=3

== system ScriptDemo/Delete/delUselessLine/Before ==
  In1 : Inport
  In2 : Inport  Port=2
  In3 : Inport  Port=3
  wires:
  In1/1 -> ?
  In2/1 -> ?
  In3/1 -> ?

== system ScriptDemo/Delete/delUselessPort/After ==
  note: <模型信息: After>
      |
      |
      | 【输入端口】
      | In2
      |
      | 【输出端口】
      | Outport1
      |
      | 【标定量】
      | 无标定量
      |
      | 创建时间: 2025-05-07 16:47:44
  In2 : Inport
  Constant : Constant
  Goto : Goto
  Outport1 : Outport
  wires:
  In2/1 -> Goto/1
  Constant/1 -> Outport1/1

== system ScriptDemo/Delete/delUselessPort/After1 ==
  In1 : Inport
  Ground : Ground
  Terminator : Terminator
  Outport : Outport
  wires:
  In1/1 -> Terminator/1
  Ground/1 -> Outport/1

== system ScriptDemo/Delete/delUselessPort/Before ==
  In1 : Inport
  In2 : Inport  Port=2
  In3 : Inport  Port=3
  Constant : Constant
  Goto : Goto
  Ground : Ground
  Terminator : Terminator
  Outport : Outport
  Outport1 : Outport  Port=2
  Outport2 : Outport  Port=3
  wires:
  In1/1 -> Terminator/1
  In2/1 -> Goto/1
  In3/1 -> ?
  Ground/1 -> Outport/1
  ? -> Outport2/1
  Constant/1 -> Outport1/1

== system ScriptDemo/Find/findModBkConnected/Before ==
  note: % 目的: 为输出端口创建debug 及对应的输入模块
      | [cnt] = createDebug(gcs)
  sTmRefriVlvCtrl_X_s32CEXVPosReqIn : Inport  OutDataTypeStr=single
  sTmRefriVlvCtrl_X_s32EEXVPosReqIn : Inport  Port=2  OutDataTypeStr=single
  sTmRefriVlvCtrl_X_s32BEXVPosReqIn : Inport  Port=3  OutDataTypeStr=single
  yTmRefriVlvCtrl_B_HpcCexvMovEnableIn : Inport  Port=4  OutDataTypeStr=boolean
  sTmRefriVlvCtrl_Z_u8CEXVInitStateIn : Inport  Port=5  OutDataTypeStr=uint8
  yTmRefriVlvCtrl_B_CexvCalibReqIn : Inport  Port=6  OutDataTypeStr=boolean
  yTmRefriVlvCtrl_B_HpcEexvMovEnableIn : Inport  Port=7  OutDataTypeStr=boolean
  sTmRefriVlvCtrl_Z_u8EEXVInitStateIn : Inport  Port=8  OutDataTypeStr=uint8
  yTmRefriVlvCtrl_B_EexvCalibReqIn : Inport  Port=9  OutDataTypeStr=boolean
  yTmRefriVlvCtrl_B_HpcBexvMovEnableIn : Inport  Port=10  OutDataTypeStr=boolean
  sTmRefriVlvCtrl_Z_u8BEXVInitStateIn : Inport  Port=11  OutDataTypeStr=uint8
  yTmRefriVlvCtrl_B_BexvCalibReqIn : Inport  Port=12  OutDataTypeStr=boolean
  sTmRefriVlvCtrl_X_s32SM3BexvMaxPosIn : Inport  Port=13  OutDataTypeStr=single
  yTmRefriVlvCtrl_B_EvapBattTLimBexvEnaIn : Inport  Port=14  OutDataTypeStr=boolean
  sTmRefriVlvCtrl_D_u8EexvRefriSwitchStIn : Inport  Port=15  OutDataTypeStr=uint8
  sTmRefriVlvCtrl_D_u8CexvRefriSwitchStIn : Inport  Port=16  OutDataTypeStr=uint8
  sTmRefriVlvCtrl_D_u8BexvRefriSwitchStIn : Inport  Port=17  OutDataTypeStr=uint8
  OutDebug : PCMULib/Interface/OutdebugRvs  SWI=cTmRefriVlvCtrl_X_s32CEXVPosReq_sw  DBI=cTmRefriVlvCtrl_X_s32CEXVPosReq_db
      settings: SourceProductName=PCMULib
  OutDebug1 : PCMULib/Interface/OutdebugRvs  SWI=cTmRefriVlvCtrl_X_s32EEXVPosReq_sw  DBI=cTmRefriVlvCtrl_X_s32EEXVPosReq_db
      settings: SourceProductName=PCMULib
  OutDebug10 : PCMULib/Interface/OutdebugRvs  SWI=cTmRefriVlvCtrl_Z_u8BEXVInitState_sw  DBI=cTmRefriVlvCtrl_Z_u8BEXVInitState_db
      settings: SourceProductName=PCMULib
  OutDebug11 : PCMULib/Interface/OutdebugRvs  SWI=cTmRefriVlvCtrl_B_BexvCalibReq_sw  DBI=cTmRefriVlvCtrl_B_BexvCalibReq_db
      settings: SourceProductName=PCMULib
  OutDebug12 : PCMULib/Interface/OutdebugRvs  SWI=cTmRefriVlvCtrl_X_s32SM3BexvMaxPos_sw  DBI=cTmRefriVlvCtrl_X_s32SM3BexvMaxPos_db
      settings: SourceProductName=PCMULib
  OutDebug13 : PCMULib/Interface/OutdebugRvs  SWI=cTmRefriVlvCtrl_B_EvapBattTLimBexvEna_sw  DBI=cTmRefriVlvCtrl_B_EvapBattTLimBexvEna_db
      settings: SourceProductName=PCMULib
  OutDebug14 : PCMULib/Interface/OutdebugRvs  SWI=cTmRefriVlvCtrl_D_u8EexvRefriSwitchSt_sw  DBI=cTmRefriVlvCtrl_D_u8EexvRefriSwitchSt_db
      settings: SourceProductName=PCMULib
  OutDebug15 : PCMULib/Interface/OutdebugRvs  SWI=cTmRefriVlvCtrl_D_u8CexvRefriSwitchSt_sw  DBI=cTmRefriVlvCtrl_D_u8CexvRefriSwitchSt_db
      settings: SourceProductName=PCMULib
  OutDebug16 : PCMULib/Interface/OutdebugRvs  SWI=cTmRefriVlvCtrl_D_u8BexvRefriSwitchSt_sw  DBI=cTmRefriVlvCtrl_D_u8BexvRefriSwitchSt_db
      settings: SourceProductName=PCMULib
  OutDebug2 : PCMULib/Interface/OutdebugRvs  SWI=cTmRefriVlvCtrl_X_s32BEXVPosReq_sw  DBI=cTmRefriVlvCtrl_X_s32BEXVPosReq_db
      settings: SourceProductName=PCMULib
  OutDebug3 : PCMULib/Interface/OutdebugRvs  SWI=cTmRefriVlvCtrl_B_HpcCexvMovEnable_sw  DBI=cTmRefriVlvCtrl_B_HpcCexvMovEnable_db
      settings: SourceProductName=PCMULib
  OutDebug4 : PCMULib/Interface/OutdebugRvs  SWI=cTmRefriVlvCtrl_Z_u8CEXVInitState_sw  DBI=cTmRefriVlvCtrl_Z_u8CEXVInitState_db
      settings: SourceProductName=PCMULib
  OutDebug5 : PCMULib/Interface/OutdebugRvs  SWI=cTmRefriVlvCtrl_B_CexvCalibReq_sw  DBI=cTmRefriVlvCtrl_B_CexvCalibReq_db
      settings: SourceProductName=PCMULib
  OutDebug6 : PCMULib/Interface/OutdebugRvs  SWI=cTmRefriVlvCtrl_B_HpcEexvMovEnable_sw  DBI=cTmRefriVlvCtrl_B_HpcEexvMovEnable_db
      settings: SourceProductName=PCMULib
  OutDebug7 : PCMULib/Interface/OutdebugRvs  SWI=cTmRefriVlvCtrl_Z_u8EEXVInitState_sw  DBI=cTmRefriVlvCtrl_Z_u8EEXVInitState_db
      settings: SourceProductName=PCMULib
  OutDebug8 : PCMULib/Interface/OutdebugRvs  SWI=cTmRefriVlvCtrl_B_EexvCalibReq_sw  DBI=cTmRefriVlvCtrl_B_EexvCalibReq_db
      settings: SourceProductName=PCMULib
  OutDebug9 : PCMULib/Interface/OutdebugRvs  SWI=cTmRefriVlvCtrl_B_HpcBexvMovEnable_sw  DBI=cTmRefriVlvCtrl_B_HpcBexvMovEnable_db
      settings: SourceProductName=PCMULib
  sTmRefriVlvCtrl_X_s32CEXVPosReq : Outport  OutDataTypeStr=single
  sTmRefriVlvCtrl_X_s32EEXVPosReq : Outport  Port=2  OutDataTypeStr=single
  sTmRefriVlvCtrl_X_s32BEXVPosReq : Outport  Port=3  OutDataTypeStr=single
  yTmRefriVlvCtrl_B_HpcCexvMovEnable : Outport  Port=4  OutDataTypeStr=boolean
  sTmRefriVlvCtrl_Z_u8CEXVInitState : Outport  Port=5  OutDataTypeStr=uint8
  yTmRefriVlvCtrl_B_CexvCalibReq : Outport  Port=6  OutDataTypeStr=boolean
  yTmRefriVlvCtrl_B_HpcEexvMovEnable : Outport  Port=7  OutDataTypeStr=boolean
  sTmRefriVlvCtrl_Z_u8EEXVInitState : Outport  Port=8  OutDataTypeStr=uint8
  yTmRefriVlvCtrl_B_EexvCalibReq : Outport  Port=9  OutDataTypeStr=boolean
  yTmRefriVlvCtrl_B_HpcBexvMovEnable : Outport  Port=10  OutDataTypeStr=boolean
  sTmRefriVlvCtrl_Z_u8BEXVInitState : Outport  Port=11  OutDataTypeStr=uint8
  yTmRefriVlvCtrl_B_BexvCalibReq : Outport  Port=12  OutDataTypeStr=boolean
  sTmRefriVlvCtrl_X_s32SM3BexvMaxPos : Outport  Port=13  OutDataTypeStr=single
  yTmRefriVlvCtrl_B_EvapBattTLimBexvEna : Outport  Port=14  OutDataTypeStr=boolean
  sTmRefriVlvCtrl_D_u8EexvRefriSwitchSt : Outport  Port=15  OutDataTypeStr=uint8
  sTmRefriVlvCtrl_D_u8CexvRefriSwitchSt : Outport  Port=16  OutDataTypeStr=uint8
  sTmRefriVlvCtrl_D_u8BexvRefriSwitchSt : Outport  Port=17  OutDataTypeStr=uint8
  wires:
  sTmRefriVlvCtrl_X_s32SM3BexvMaxPosIn/1 -> OutDebug12/1
  OutDebug12/1 -> sTmRefriVlvCtrl_X_s32SM3BexvMaxPos/1
  sTmRefriVlvCtrl_X_s32BEXVPosReqIn/1 -> OutDebug2/1
  OutDebug2/1 -> sTmRefriVlvCtrl_X_s32BEXVPosReq/1
  OutDebug16/1 -> sTmRefriVlvCtrl_D_u8BexvRefriSwitchSt/1
  sTmRefriVlvCtrl_D_u8EexvRefriSwitchStIn/1 -> OutDebug14/1
  OutDebug5/1 -> yTmRefriVlvCtrl_B_CexvCalibReq/1
  OutDebug3/1 -> yTmRefriVlvCtrl_B_HpcCexvMovEnable/1
  sTmRefriVlvCtrl_Z_u8CEXVInitStateIn/1 -> OutDebug4/1
  OutDebug4/1 -> sTmRefriVlvCtrl_Z_u8CEXVInitState/1
  sTmRefriVlvCtrl_D_u8BexvRefriSwitchStIn/1 -> OutDebug16/1
  OutDebug1/1 -> sTmRefriVlvCtrl_X_s32EEXVPosReq/1
  OutDebug14/1 -> sTmRefriVlvCtrl_D_u8EexvRefriSwitchSt/1
  yTmRefriVlvCtrl_B_CexvCalibReqIn/1 -> OutDebug5/1
  sTmRefriVlvCtrl_X_s32EEXVPosReqIn/1 -> OutDebug1/1
  yTmRefriVlvCtrl_B_HpcCexvMovEnableIn/1 -> OutDebug3/1
  yTmRefriVlvCtrl_B_EvapBattTLimBexvEnaIn/1 -> OutDebug13/1
  OutDebug13/1 -> yTmRefriVlvCtrl_B_EvapBattTLimBexvEna/1
  sTmRefriVlvCtrl_Z_u8BEXVInitStateIn/1 -> OutDebug10/1
  OutDebug10/1 -> sTmRefriVlvCtrl_Z_u8BEXVInitState/1
  sTmRefriVlvCtrl_D_u8CexvRefriSwitchStIn/1 -> OutDebug15/1
  OutDebug15/1 -> sTmRefriVlvCtrl_D_u8CexvRefriSwitchSt/1
  OutDebug/1 -> sTmRefriVlvCtrl_X_s32CEXVPosReq/1
  OutDebug7/1 -> sTmRefriVlvCtrl_Z_u8EEXVInitState/1
  OutDebug8/1 -> yTmRefriVlvCtrl_B_EexvCalibReq/1
  yTmRefriVlvCtrl_B_EexvCalibReqIn/1 -> OutDebug8/1
  sTmRefriVlvCtrl_X_s32CEXVPosReqIn/1 -> OutDebug/1
  OutDebug6/1 -> yTmRefriVlvCtrl_B_HpcEexvMovEnable/1
  yTmRefriVlvCtrl_B_HpcEexvMovEnableIn/1 -> OutDebug6/1
  sTmRefriVlvCtrl_Z_u8EEXVInitStateIn/1 -> OutDebug7/1
  yTmRefriVlvCtrl_B_HpcBexvMovEnableIn/1 -> OutDebug9/1
  OutDebug9/1 -> yTmRefriVlvCtrl_B_HpcBexvMovEnable/1
  yTmRefriVlvCtrl_B_BexvCalibReqIn/1 -> OutDebug11/1
  OutDebug11/1 -> yTmRefriVlvCtrl_B_BexvCalibReq/1
